simulink model "dual_arm_control"  (Simulink 7.8)
settings: Solver=ode1  StartTime=0.0  StopTime=inf  FixedStep=0.001  RelTol=1e-3
undefined symbols (not defined in the file): HIL
libraries: quarc_library x48, simulink x26, dspmtrx3 x5
(part 2 of 2)

== system dual_arm_control/Right Arm/contoller 22 ==
  qd : Inport
  q : Inport  Port=2
  en : Inport  Port=3
  Constant : Constant  Value=20
  Constant1 : Constant  Value=5e9
  Derivative3 : Derivative
  Derivative4 : Derivative
  Derivative5 : Derivative
  Memory3 : Memory  X0="[-0.0039    0.0394    0.0222   -0.2171]'"
  slotine's adaptive : MATLAB Function  TreatAsAtomicUnit=on
  tau : Outport
  ahat : Outport  Port=2
  wires:
  Derivative4/1 -> slotine's adaptive/6(qddotdot)
  Derivative5/1 -> slotine's adaptive/8(qdot)
  Derivative3/1 -> Derivative4/1, slotine's adaptive/5(qddot)
  slotine's adaptive/2(ahat) -> Memory3/1, ahat/1
  Memory3/1 -> slotine's adaptive/9(ahat_)
  Constant/1 -> slotine's adaptive/2(lambda)
  Constant1/1 -> slotine's adaptive/3(gamma)
  qd/1 -> slotine's adaptive/4(qd), Derivative3/1
  q/1 -> slotine's adaptive/7(q), Derivative5/1
  slotine's adaptive/1(tau) -> tau/1
  en/1 -> slotine's adaptive/1(en)

== system dual_arm_control/Right Arm/controller 21 ==
  qd : Inport
  q : Inport  Port=2
  en : Inport  Port=3
  Constant : Constant  Value=60
  Constant1 : Constant  Value=1e8
  Derivative3 : Derivative
  Derivative4 : Derivative
  Derivative5 : Derivative
  Memory3 : Memory  X0="[3.3914    0.1816    0.3172    0.1486   -5.6249]'"
  slotine's adaptive : MATLAB Function  TreatAsAtomicUnit=on
  tau : Outport
  ahat : Outport  Port=2
  wires:
  Derivative4/1 -> slotine's adaptive/6(qddotdot)
  Derivative5/1 -> slotine's adaptive/8(qdot)
  Derivative3/1 -> Derivative4/1, slotine's adaptive/5(qddot)
  slotine's adaptive/2(ahat) -> Memory3/1, ahat/1
  Memory3/1 -> slotine's adaptive/9(ahat_)
  Constant/1 -> slotine's adaptive/2(lambda)
  Constant1/1 -> slotine's adaptive/3(gamma)
  qd/1 -> slotine's adaptive/4(qd), Derivative3/1
  q/1 -> slotine's adaptive/7(q), Derivative5/1
  slotine's adaptive/1(tau) -> tau/1
  en/1 -> slotine's adaptive/1(en)

== system dual_arm_control/Right Arm/controller 23 ==
  qd : Inport
  q : Inport  Port=2
  en : Inport  Port=3
  Constant : Constant  Value=50
  Constant1 : Constant  Value=1e6
  Derivative3 : Derivative
  Derivative4 : Derivative
  Derivative5 : Derivative
  Memory3 : Memory  X0="[3.3916    0.1811    0.0907   -5.6122]'"
  slotine's adaptive : MATLAB Function  TreatAsAtomicUnit=on
  tau : Outport
  ahat : Outport  Port=2
  wires:
  Derivative4/1 -> slotine's adaptive/6(qddotdot)
  Derivative5/1 -> slotine's adaptive/8(qdot)
  Derivative3/1 -> Derivative4/1, slotine's adaptive/5(qddot)
  slotine's adaptive/2(ahat) -> Memory3/1, ahat/1
  Memory3/1 -> slotine's adaptive/9(ahat_)
  Constant/1 -> slotine's adaptive/2(lambda)
  Constant1/1 -> slotine's adaptive/3(gamma)
  qd/1 -> slotine's adaptive/4(qd), Derivative3/1
  q/1 -> slotine's adaptive/7(q), Derivative5/1
  slotine's adaptive/1(tau) -> tau/1
  en/1 -> slotine's adaptive/1(en)

== system dual_arm_control/Right Arm/controller 24 ==
  qd : Inport
  q : Inport  Port=2
  en : Inport  Port=3
  Constant : Constant  Value=50
  Constant1 : Constant  Value=1e6
  Derivative3 : Derivative
  Derivative4 : Derivative
  Derivative5 : Derivative
  Memory3 : Memory  X0="[0.0008    0.0273    0.0390   -0.0832]'"
  slotine's adaptive : MATLAB Function  TreatAsAtomicUnit=on
  tau : Outport
  ahat : Outport  Port=2
  wires:
  Derivative4/1 -> slotine's adaptive/6(qddotdot)
  Derivative5/1 -> slotine's adaptive/8(qdot)
  Derivative3/1 -> Derivative4/1, slotine's adaptive/5(qddot)
  slotine's adaptive/2(ahat) -> Memory3/1, ahat/1
  Memory3/1 -> slotine's adaptive/9(ahat_)
  Constant/1 -> slotine's adaptive/2(lambda)
  Constant1/1 -> slotine's adaptive/3(gamma)
  qd/1 -> slotine's adaptive/4(qd), Derivative3/1
  q/1 -> slotine's adaptive/7(q), Derivative5/1
  slotine's adaptive/1(tau) -> tau/1
  en/1 -> slotine's adaptive/1(en)

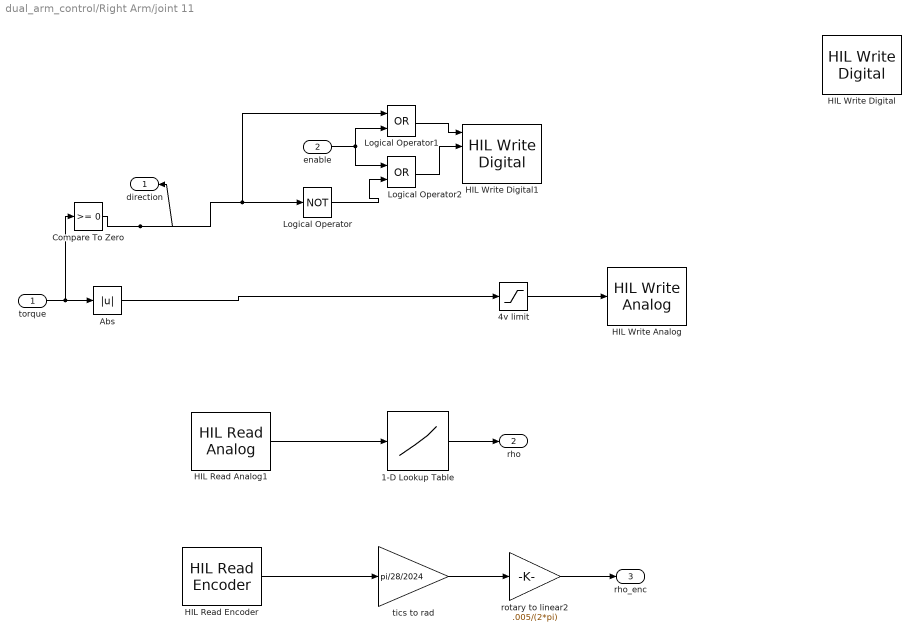
== system dual_arm_control/Right Arm/joint 11 ==
  torque : Inport
  enable : Inport  Port=2
  1-D Lookup Table : Lookup_n-D  NumberOfTableDimensions=1  BreakpointsForDimension1="[.147 .227 .277 .376 .459 .597  .742  .929  1.132  1.36 1.55   1.78  2.078 2.43 2.768  3.016   3.233  3.49  3.78  4.03 4.28]"  Table="[.04 .0375 .0357 .033 .031 .0286 .026  .022  .018  .015  .013  .01  .0088  .0077  .006   .005  .004  .003  .002  .001 0]"  RndMeth=Simplest  InputSameDT=on
  4v limit : Saturate  UpperLimit=4  LowerLimit=0
  Abs : Abs
  Compare To Zero : simulink/Logic and Bit Operations/Compare To Zero  relop=>=  OutDataTypeStr=boolean
  HIL Read Analog1 : quarc_library/Data Acquisition/Generic/Immediate I//O/HIL Read Analog  object_name=HIL-2  channels=[4]  sample_time=qc_get_step_size  active=on  vector_output=off
  HIL Read Encoder : quarc_library/Data Acquisition/Generic/Immediate I//O/HIL Read Encoder  object_name=HIL-2  channels=[0]  sample_time=qc_get_step_size  active=on  vector_output=off  data_type_mode=Inherit via back propagation  data_type=double
  HIL Write Analog : quarc_library/Data Acquisition/Generic/Immediate I//O/HIL Write Analog  object_name=HIL-1  channels=[0]  sample_time=-1  active=off  vector_input=off
  HIL Write Digital : quarc_library/Data Acquisition/Generic/Immediate I//O/HIL Write Digital  object_name=HIL-1  channels=[0:3]  sample_time=-1  active=off  vector_input=off
  HIL Write Digital1 : quarc_library/Data Acquisition/Generic/Immediate I//O/HIL Write Digital  object_name=HIL-1  channels=[40:43]  sample_time=-1  active=off  vector_input=off
  Logical Operator : Logic  Operator=NOT  AllPortsSameDT=off  OutDataTypeStr=boolean
  Logical Operator1 : Logic  Operator=OR  AllPortsSameDT=off  OutDataTypeStr=boolean
  Logical Operator2 : Logic  Operator=OR  AllPortsSameDT=off  OutDataTypeStr=boolean
  rotary to linear2 : Gain  Gain=.005/(2*pi)
  tics to rad : Gain  Gain=pi/28/2024
  direction : Outport
  rho : Outport  Port=2
  rho_enc : Outport  Port=3
  wires:
  4v limit/1 -> HIL Write Analog/1
  Compare To Zero/1 -> direction/1, Logical Operator/1, Logical Operator1/1
  Abs/1 -> 4v limit/1
  torque/1 -> Abs/1, Compare To Zero/1
  HIL Read Analog1/1 -> 1-D Lookup Table/1
  HIL Read Encoder/1 -> tics to rad/1
  Logical Operator/1 -> Logical Operator2/2
  enable/1 -> Logical Operator1/2, Logical Operator2/1
  Logical Operator1/1 -> HIL Write Digital1/1
  Logical Operator2/1 -> HIL Write Digital1/2
  1-D Lookup Table/1 -> rho/1
  tics to rad/1 -> rotary to linear2/1
  rotary to linear2/1 -> rho_enc/1

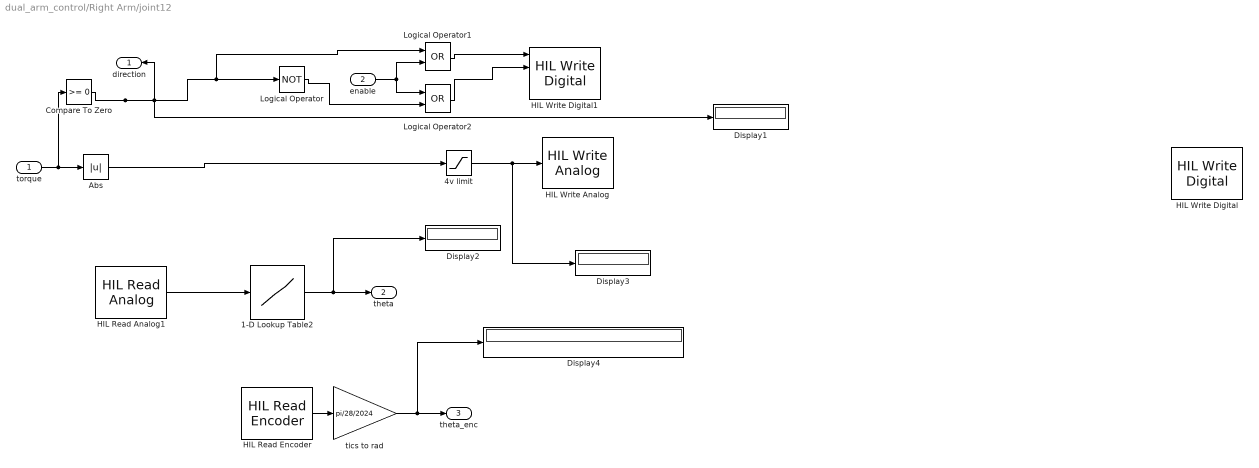
== system dual_arm_control/Right Arm/joint12 ==
  torque : Inport
  enable : Inport  Port=2
  1-D Lookup Table2 : Lookup_n-D  NumberOfTableDimensions=1  BreakpointsForDimension1=[.78 1.64 2.51 3.40 4.27]  Table=[2 1 0 -1 -2]  RndMeth=Simplest  InputSameDT=on
  4v limit : Saturate  UpperLimit=4  LowerLimit=0
  Abs : Abs
  Compare To Zero : simulink/Logic and Bit Operations/Compare To Zero  relop=>=  OutDataTypeStr=boolean
  Display{1..4} (4 alike) : Display
  HIL Read Analog1 : quarc_library/Data Acquisition/Generic/Immediate I//O/HIL Read Analog  object_name=HIL-1  channels=[3]  sample_time=qc_get_step_size  active=on  vector_output=off
  HIL Read Encoder : quarc_library/Data Acquisition/Generic/Immediate I//O/HIL Read Encoder  object_name=HIL-2  channels=[1]  sample_time=qc_get_step_size  active=on  vector_output=off  data_type_mode=Inherit via back propagation  data_type=double
  HIL Write Analog : quarc_library/Data Acquisition/Generic/Immediate I//O/HIL Write Analog  object_name=HIL-1  channels=[1]  sample_time=-1  active=off  vector_input=off
  HIL Write Digital : quarc_library/Data Acquisition/Generic/Immediate I//O/HIL Write Digital  object_name=HIL-1  channels=[4:7]  sample_time=-1  active=off  vector_input=off
  HIL Write Digital1 : quarc_library/Data Acquisition/Generic/Immediate I//O/HIL Write Digital  object_name=HIL-1  channels=[44:47]  sample_time=-1  active=off  vector_input=off
  Logical Operator : Logic  Operator=NOT  AllPortsSameDT=off  OutDataTypeStr=boolean
  Logical Operator1 : Logic  Operator=OR  AllPortsSameDT=off  OutDataTypeStr=boolean
  Logical Operator2 : Logic  Operator=OR  AllPortsSameDT=off  OutDataTypeStr=boolean
  tics to rad : Gain  Gain=pi/28/2024
  direction : Outport
  theta : Outport  Port=2
  theta_enc : Outport  Port=3
  wires:
  4v limit/1 -> HIL Write Analog/1, Display3/1
  Compare To Zero/1 -> Logical Operator/1, Logical Operator1/1, direction/1, Display1/1
  Abs/1 -> 4v limit/1
  torque/1 -> Abs/1, Compare To Zero/1
  HIL Read Analog1/1 -> 1-D Lookup Table2/1
  HIL Read Encoder/1 -> tics to rad/1
  Logical Operator1/1 -> HIL Write Digital1/1
  Logical Operator2/1 -> HIL Write Digital1/2
  Logical Operator/1 -> Logical Operator2/2
  enable/1 -> Logical Operator1/2, Logical Operator2/1
  tics to rad/1 -> theta_enc/1, Display4/1
  1-D Lookup Table2/1 -> Display2/1, theta/1

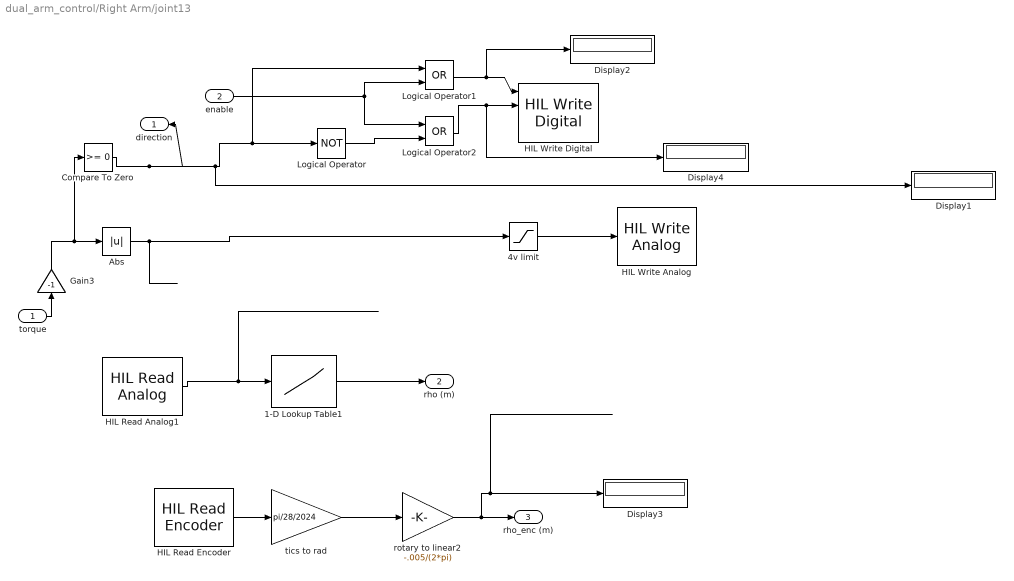
== system dual_arm_control/Right Arm/joint13 ==
  torque : Inport
  enable : Inport  Port=2
  1-D Lookup Table1 : Lookup_n-D  NumberOfTableDimensions=1  BreakpointsForDimension1="[.255 .369 .511 .661 .806 .966 1.075  1.274 1.456 1.643 1.858 2.075 2.328 2.50 2.753 3.011 3.23 3.39 4 4.191 4.384 4.628 4.84 4.963]"  Table=[0 .004 .0067 .0094 .012 .015 .017 .0199 .022 .0245 .0263 .0279 .0287 .0294 .030 .0315 .032 .034 .0357 .0365 .0373 .0385 .039 .04]+.001  RndMeth=Simplest  InputSameDT=on
  4v limit : Saturate  UpperLimit=4  LowerLimit=0
  Abs : Abs
  Compare To Zero : simulink/Logic and Bit Operations/Compare To Zero  relop=>=  OutDataTypeStr=boolean
  Display{1..4} (4 alike) : Display
  Gain3 : Gain  Gain=-1
  HIL Read Analog1 : quarc_library/Data Acquisition/Generic/Immediate I//O/HIL Read Analog  object_name=HIL-2  channels=[5]  sample_time=qc_get_step_size  active=on  vector_output=off
  HIL Read Encoder : quarc_library/Data Acquisition/Generic/Immediate I//O/HIL Read Encoder  object_name=HIL-2  channels=[2]  sample_time=qc_get_step_size  active=on  vector_output=off  data_type_mode=Inherit via back propagation  data_type=double
  HIL Write Analog : quarc_library/Data Acquisition/Generic/Immediate I//O/HIL Write Analog  object_name=HIL-1  channels=[2]  sample_time=-1  active=off  vector_input=off
  HIL Write Digital : quarc_library/Data Acquisition/Generic/Immediate I//O/HIL Write Digital  object_name=HIL-1  channels=[8:11]  sample_time=-1  active=off  vector_input=off
  Logical Operator : Logic  Operator=NOT  AllPortsSameDT=off  OutDataTypeStr=boolean
  Logical Operator1 : Logic  Operator=OR  AllPortsSameDT=off  OutDataTypeStr=boolean
  Logical Operator2 : Logic  Operator=OR  AllPortsSameDT=off  OutDataTypeStr=boolean
  rotary to linear2 : Gain  Gain=-.005/(2*pi)
  tics to rad : Gain  Gain=pi/28/2024
  direction : Outport
  rho (m) : Outport  Port=2
  rho_enc (m) : Outport  Port=3
  wires:
  4v limit/1 -> HIL Write Analog/1
  Compare To Zero/1 -> Logical Operator/1, Logical Operator1/1, Display1/1, direction/1
  Abs/1 -> 4v limit/1
  torque/1 -> Gain3/1
  HIL Read Analog1/1 -> 1-D Lookup Table1/1
  HIL Read Encoder/1 -> tics to rad/1
  Logical Operator/1 -> Logical Operator2/2
  Logical Operator2/1 -> HIL Write Digital/2, Display4/1
  Logical Operator1/1 -> HIL Write Digital/1, Display2/1
  enable/1 -> Logical Operator1/2, Logical Operator2/1
  1-D Lookup Table1/1 -> rho (m)/1
  tics to rad/1 -> rotary to linear2/1
  rotary to linear2/1 -> rho_enc (m)/1, Display3/1
  Gain3/1 -> Abs/1, Compare To Zero/1

== system dual_arm_control/Subsystem2/E1-1 ==
  Gain : Gain  Gain=pi
  HIL Read Analog : quarc_library/Data Acquisition/Generic/Immediate I//O/HIL Read Analog  object_name=HIL-2  channels=[0]  sample_time=qc_get_step_size  active=on  vector_output=off
  Out1 : Outport
  wires:
  HIL Read Analog/1 -> Gain/1
  Gain/1 -> Out1/1

== system dual_arm_control/Subsystem2/E1-2 ==
  Gain : Gain  Gain=pi
  HIL Read Analog : quarc_library/Data Acquisition/Generic/Immediate I//O/HIL Read Analog  object_name=HIL-2  channels=[1]  sample_time=qc_get_step_size  active=on  vector_output=off
  Out1 : Outport
  wires:
  HIL Read Analog/1 -> Gain/1
  Gain/1 -> Out1/1

== system dual_arm_control/Subsystem2/Subsystem ==
  DIR_1 : Inport
  EN_1 : Inport  Port=2
  PWM_1 : Inport  Port=3
  DIR_2 : Inport  Port=4
  EN_2 : Inport  Port=5
  PWM_2 : Inport  Port=6
  Constant3 : Constant
  Display : Display
  Display1 : Display
  E1-1 : Subsystem
  E1-2 : Subsystem
  E1-A : Subsystem
  Scope : Scope
  Scope1 : Scope
  wires:
  Constant3/1 -> E1-A/4(STBY)
  E1-1/1(IN1) -> E1-A/1(BIN1)
  E1-1/2(IN2) -> E1-A/2(BIN2)
  E1-1/3(PWM) -> E1-A/3(PWMB), Display/1, Scope/1
  E1-2/1(IN1) -> E1-A/5(AIN1)
  E1-2/2(IN2) -> E1-A/6(AIN2)
  E1-2/3(PWM) -> E1-A/7(PWMA), Display1/1, Scope1/1
  DIR_1/1 -> E1-1/1(DIR)
  EN_1/1 -> E1-1/2(EN)
  PWM_1/1 -> E1-1/3(DC)
  DIR_2/1 -> E1-2/1(DIR)
  EN_2/1 -> E1-2/2(EN)
  PWM_2/1 -> E1-2/3(DC)

== system dual_arm_control/IK_L/from omni/haptic gravity compensation ==
  position : Inport
  boundary force : Inport  Port=2
  status : Inport  Port=3
  Constant : Constant  Value=[0 0 .5]
  Derivative : Derivative
  Display1 : Display
  Display4 : Display
  Gain : Gain  Gain=-.030*diag([1 1 1])  Multiplication=Matrix(K*u)
  Gain1 : Gain  Gain=-.35*diag([1 1 1])  Multiplication=Matrix(K*u)
  Multiport Switch : MultiPortSwitch  Inputs=7  zeroidx=off
  Sum : Sum  Inputs=|+++++
  Sum1 : Sum  Inputs=|++
  force : Outport
  wires:
  Derivative/1 -> Gain/1
  Sum/1 -> force/1
  position/1 -> Derivative/1, Gain1/1
  Constant/1 -> Sum/4
  status/1 -> [status]
  Gain/1 -> Sum1/1
  Multiport Switch/1 -> Sum/1, Display4/1
  [status] -> Multiport Switch/1, Display1/1
  Sum1/1 -> Sum/5
  Gain1/1 -> Multiport Switch/7
  boundary force/1 -> Multiport Switch/8

== system dual_arm_control/IK_L/phantom/haptic gravity compensation ==
  position : Inport
  boundary force : Inport  Port=2
  status : Inport  Port=3
  Constant : Constant  Value=[0 0 .92]
  Derivative : Derivative
  Display1 : Display
  Display2 : Display
  Gain : Gain  Gain=-.1*diag([1 1 1])  Multiplication=Matrix(K*u)
  Gain1 : Gain  Gain=-.8*diag([1 1 1])  Multiplication=Matrix(K*u)
  Multiport Switch : MultiPortSwitch  Inputs=7  zeroidx=off
  Sum : Sum  Inputs=|+++++
  Sum1 : Sum  Inputs=|++
  force : Outport
  wires:
  Derivative/1 -> Gain/1
  Sum/1 -> force/1
  position/1 -> Derivative/1, Gain1/1
  Constant/1 -> Sum/4
  status/1 -> [status]
  Gain/1 -> Sum1/1
  Multiport Switch/1 -> Sum/1
  [status] -> Multiport Switch/1, Display1/1
  Sum1/1 -> Sum/5
  Gain1/1 -> Multiport Switch/7
  boundary force/1 -> Multiport Switch/8

== system dual_arm_control/Subsystem2/Subsystem/E1-1 ==
  DIR : Inport
  EN : Inport  Port=2
  DC : Inport  Port=3
  Logical Operator : Logic  AllPortsSameDT=off  OutDataTypeStr=boolean
  Logical Operator1 : Logic  AllPortsSameDT=off  OutDataTypeStr=boolean
  Logical Operator2 : Logic  Operator=NOT  AllPortsSameDT=off  OutDataTypeStr=boolean
  pwm generator : Subsystem
  IN1 : Outport
  IN2 : Outport  Port=2
  PWM : Outport  Port=3
  wires:
  Logical Operator2/1 -> Logical Operator/1
  DIR/1 -> Logical Operator2/1, Logical Operator1/1
  EN/1 -> Logical Operator/2, Logical Operator1/2
  Logical Operator/1 -> IN1/1
  Logical Operator1/1 -> IN2/1
  DC/1 -> pwm generator/1(In1)
  pwm generator/1(Out1) -> PWM/1

== system dual_arm_control/Subsystem2/Subsystem/E1-2 ==
  DIR : Inport
  EN : Inport  Port=2
  DC : Inport  Port=3
  Logical Operator : Logic  AllPortsSameDT=off  OutDataTypeStr=boolean
  Logical Operator1 : Logic  AllPortsSameDT=off  OutDataTypeStr=boolean
  Logical Operator2 : Logic  Operator=NOT  AllPortsSameDT=off  OutDataTypeStr=boolean
  pwm generator : Subsystem
  IN1 : Outport
  IN2 : Outport  Port=2
  PWM : Outport  Port=3
  wires:
  Logical Operator2/1 -> Logical Operator/1
  DIR/1 -> Logical Operator2/1, Logical Operator1/1
  EN/1 -> Logical Operator/2, Logical Operator1/2
  Logical Operator/1 -> IN1/1
  Logical Operator1/1 -> IN2/1
  DC/1 -> pwm generator/1(In1)
  pwm generator/1(Out1) -> PWM/1

== system dual_arm_control/Subsystem2/Subsystem/E1-A ==
  BIN1 : Inport
  BIN2 : Inport  Port=2
  PWMB : Inport  Port=3
  STBY : Inport  Port=4
  AIN1 : Inport  Port=5
  AIN2 : Inport  Port=6
  PWMA : Inport  Port=7
  HIL Write Digital : quarc_library/Data Acquisition/Generic/Immediate I//O/HIL Write Digital  object_name=HIL-2  channels=[44]  sample_time=-1  active=off  vector_input=off
  HIL Write Digital1 : quarc_library/Data Acquisition/Generic/Immediate I//O/HIL Write Digital  object_name=HIL-2  channels=[43]  sample_time=-1  active=off  vector_input=off
  HIL Write Digital2 : quarc_library/Data Acquisition/Generic/Immediate I//O/HIL Write Digital  object_name=HIL-2  channels=[42]  sample_time=-1  active=off  vector_input=off
  HIL Write Digital3 : quarc_library/Data Acquisition/Generic/Immediate I//O/HIL Write Digital  object_name=HIL-2  channels=[41]  sample_time=-1  active=off  vector_input=off
  HIL Write Digital4 : quarc_library/Data Acquisition/Generic/Immediate I//O/HIL Write Digital  object_name=HIL-2  channels=[45]  sample_time=-1  active=off  vector_input=off
  HIL Write Digital5 : quarc_library/Data Acquisition/Generic/Immediate I//O/HIL Write Digital  object_name=HIL-2  channels=[46]  sample_time=-1  active=off  vector_input=off
  HIL Write Digital6 : quarc_library/Data Acquisition/Generic/Immediate I//O/HIL Write Digital  object_name=HIL-2  channels=[47]  sample_time=-1  active=off  vector_input=off
  wires:
  BIN1/1 -> HIL Write Digital1/1
  BIN2/1 -> HIL Write Digital2/1
  PWMB/1 -> HIL Write Digital3/1
  STBY/1 -> HIL Write Digital/1
  AIN1/1 -> HIL Write Digital4/1
  AIN2/1 -> HIL Write Digital5/1
  PWMA/1 -> HIL Write Digital6/1

== system dual_arm_control/Subsystem2/Subsystem/E1-1/pwm generator ==
  In1 : Inport
  Counter Limited : simulink/Sources/Counter Limited  uplimit=10  tsamp=-1
  Gain : Gain  Gain=.1
  Relational Operator : RelationalOperator  Operator=<=  OutDataTypeStr=boolean
  Out1 : Outport
  wires:
  Counter Limited/1 -> Gain/1
  Gain/1 -> Relational Operator/1
  Relational Operator/1 -> Out1/1
  In1/1 -> Relational Operator/2

== system dual_arm_control/Subsystem2/Subsystem/E1-2/pwm generator ==
  In1 : Inport
  Counter Limited : simulink/Sources/Counter Limited  uplimit=10  tsamp=-1
  Gain : Gain  Gain=.1
  Relational Operator : RelationalOperator  Operator=<=  OutDataTypeStr=boolean
  Out1 : Outport
  wires:
  Counter Limited/1 -> Gain/1
  Gain/1 -> Relational Operator/1
  Relational Operator/1 -> Out1/1
  In1/1 -> Relational Operator/2

== matlab function Left Arm/controller 24/slotine's adaptive ==
  data: en input double; lambda input double; gamma input double; qd input double; qddot input double; qddotdot input double; q input double; tau output double; qdot input double; ahat output double; ahat_ input double
function [tau,ahat] = fcn(en,lambda,gamma,qd,qddot,qddotdot,q,qdot,ahat_)
%#codegen


qtilde=q-qd;
qtildedot=qdot-qddot;
s=qtildedot+lambda*qtilde;
Y=[qddotdot qddot sign(qdot) s ];
ahat=-.001*en/gamma*Y'*s+ahat_;
qr=qd-(ahat(end)+lambda)*qtilde;
qrdot=qddot-(ahat(end)+lambda)*qtilde;
qrdotdot=qddotdot-(ahat(end)+lambda)*qtildedot;

tau=[qrdotdot qrdot  sign(qdot) s ]*ahat;

== matlab function MATLAB Function ==
  data: ready_ input double; ready output double; status_ input double; delq_R_ input double; delq_L_ input double; status output double; delq_R output double; delq_L output double; dqin_L input double; dqin_R input double; time input double; dummy output double; qpot_R input double; qpot_L input double
function [ready,status,delq_R,delq_L,dummy] = fcn(ready_,status_,delq_R_,delq_L_,dqin_L,dqin_R,time,qpot_R,qpot_L)
%#codegen
dummy=0;
ready=ready_;
status=status_;
delq_R=delq_R_;
delq_L=delq_L_;
if time>2 && not(ready)
    
    switch status
        case 0
%             if time>2 && time<6
                if abs(qpot_L(2))<.1
                    status=1;
                end
                delq_L=[0 dqin_L(2) 0 0]';
                
%             end
        case 1
%             if time>6 && time<10
                
                if abs(qpot_L(1))<.001
                    status=2;
                end
                delq_L=[dqin_L(1) dqin_L(2) 0 0]';
                
%             end
        case 2
%             if time>10 && time<14
                
                if abs(qpot_L(3))<.001
                    status=3;
                end
                delq_L=[dqin_L(1) dqin_L(2) dqin_L(3) 0]';
                
%             end
        case 3
%             if time>14 && time<18
                if abs(qpot_R(2))<.1
                    status=4;
                end
                delq_R=[0 dqin_R(2) 0 0]';
                
%             end
        case 4
%             if time>18 && time<22
                
                if abs(qpot_R(1))<.001
                    status=5;
                end
                delq_R=[dqin_R(1) dqin_R(2) 0 0]';
                
%             end
        case 5
%             if time>22 && time<26
                
                if abs(qpot_R(3))<.001
                    status=6;

                end
                delq_R=[dqin_R(1) dqin_R(2) dqin_R(3) 0]';
                
%             end
        case 6 %match master and slave
            if time>20
                status=7;
                ready=1;
            end
    end
    
    
end

% if ready
%     delq_R=[dqin_R(1) 0 dqin_R(3) 0]';
%     delq_L=[dqin_L(1) 0 dqin_L(3) 0]';
% end

== matlab function filter/filter ==
  data: u input double; y output double; u_ input double
function y = fcn(u,u_)
%#codegen
if u>0
    a=2;
end
if abs(u-u_)<4*pi*.001
    y=u;
else
    y=u_+4*pi*.001*(u-u_)/abs(u-u_);

end

== matlab function Left Arm/controller 23/slotine's adaptive ==
  data: en input double; lambda input double; gamma input double; qd input double; qddot input double; qddotdot input double; q input double; tau output double; qdot input double; ahat output double; ahat_ input double
function [tau,ahat] = fcn(en,lambda,gamma,qd,qddot,qddotdot,q,qdot,ahat_)
%#codegen


qtilde=q-qd;
qtildedot=qdot-qddot;
s=qtildedot+lambda*qtilde;
Y=[qddotdot qddot sign(qdot) s ];
ahat=-.001*en/gamma*Y'*s+ahat_;
qr=qd-(ahat(end)+lambda)*qtilde;
qrdot=qddot-(ahat(end)+lambda)*qtilde;
qrdotdot=qddotdot-(ahat(end)+lambda)*qtildedot;

tau=[qrdotdot qrdot  sign(qdot) s ]*ahat;

== matlab function filter1/filter ==
  data: u input double; y output double; u_ input double
function y = fcn(u,u_)
%#codegen
if u>0
    a=2;
end
if abs(u-u_)<.02*.001
    y=u;
else
    y=u_+.02*.001*(u-u_)/abs(u-u_);

end

== matlab function Left Arm/contoller 22/slotine's adaptive ==
  data: en input double; lambda input double; gamma input double; qd input double; qddot input double; qddotdot input double; q input double; tau output double; qdot input double; ahat output double; ahat_ input double
function [tau,ahat] = fcn(en,lambda,gamma,qd,qddot,qddotdot,q,qdot,ahat_)
%#codegen


qtilde=q-qd;
qtildedot=qdot-qddot;
s=qtildedot+lambda*qtilde;
Y=[qddotdot qddot sign(qdot) s ];
ahat=-.001*en/gamma*Y'*s+ahat_;
qr=qd-(ahat(end)+lambda)*qtilde;
qrdot=qddot-(ahat(end)+lambda)*qtilde;
qrdotdot=qddotdot-(ahat(end)+lambda)*qtildedot;

tau=[qrdotdot qrdot  sign(qdot) s ]*ahat;

== matlab function filter2/filter ==
  data: u input double; y output double; u_ input double
function y = fcn(u,u_)
%#codegen
if u>0
    a=2;
end
if abs(u-u_)<4*pi*.001
    y=u;
else
    y=u_+4*pi*.001*(u-u_)/abs(u-u_);

end

== matlab function Left Arm/controller 21/slotine's adaptive ==
  data: en input double; lambda input double; gamma input double; qd input double; qddot input double; qddotdot input double; q input double; tau output double; qdot input double; ahat output double; ahat_ input double
function [tau,ahat] = fcn(en,lambda,gamma,qd,qddot,qddotdot,q,qdot,ahat_)
%#codegen


qtilde=q-qd;
qtildedot=qdot-qddot;
s=qtildedot+lambda*qtilde;
Y=[qddotdot qddot  sign(qdot)-1 sign(qdot)+1 s ];
ahat=-.001*en/gamma*Y'*s+ahat_;
qr=qd-(ahat(end)+lambda)*qtilde;
qrdot=qddot-(ahat(end)+lambda)*qtilde;
qrdotdot=qddotdot-(ahat(end)+lambda)*qtildedot;

tau=[qrdotdot qrdot sign(qdot)-1 sign(qdot)+1 s ]*ahat;

== matlab function filter3/filter ==
  data: u input double; y output double; u_ input double
function y = fcn(u,u_)
%#codegen
if u>0
    a=2;
end
if abs(u-u_)<.02*.001
    y=u;
else
    y=u_+.02*.001*(u-u_)/abs(u-u_);

end

== matlab function Right Arm/contoller 22/slotine's adaptive ==
  data: en input double; lambda input double; gamma input double; qd input double; qddot input double; qddotdot input double; q input double; tau output double; qdot input double; ahat output double; ahat_ input double
function [tau,ahat] = fcn(en,lambda,gamma,qd,qddot,qddotdot,q,qdot,ahat_)
%#codegen


qtilde=q-qd;
qtildedot=qdot-qddot;
s=qtildedot+lambda*qtilde;
Y=[qddotdot qddot sign(qdot) s ];
ahat=-.001*en/gamma*Y'*s+ahat_;
qr=qd-(ahat(end)+lambda)*qtilde;
qrdot=qddot-(ahat(end)+lambda)*qtilde;
qrdotdot=qddotdot-(ahat(end)+lambda)*qtildedot;

tau=[qrdotdot qrdot  sign(qdot) s ]*ahat;

== matlab function IK_L/IK_L/IK ==
  data: q_ input double; q output double; qm output double; qdot output double; p output double; pd input double; pd_d input double; F output double; k_ input double; k output double; r_ input double; r output double
function [q,qm,qdot,p,F,k,r] = fcn(q_,pd,pd_d,k_,r_)
%#codegen
kappa=1/8.5;
x=pd(1);
y=pd(2);
z=pd(3);
r=sqrt(x^2+y^2);

rho_1=q_(1);
theta_1=q_(2);
rho_2=q_(3);
%%%%%
J =...
    [ -kappa*cos(kappa*rho_1)*cos(theta_1)*(rho_1 - (rho_2+1)),   (sin(theta_1)*(cos(kappa*rho_1) - 1))/kappa + sin(kappa*rho_1)*sin(theta_1)*(rho_1 - (rho_2+1)), sin(kappa*rho_1)*cos(theta_1)
    -kappa*cos(kappa*rho_1)*sin(theta_1)*(rho_1 - (rho_2+1)), - (cos(theta_1)*(cos(kappa*rho_1) - 1))/kappa - sin(kappa*rho_1)*cos(theta_1)*(rho_1 - (rho_2+1)), sin(kappa*rho_1)*sin(theta_1)
    kappa*sin(kappa*rho_1)*(rho_1 - (rho_2+1)),                                                                                             0,              cos(kappa*rho_1)];


qdot=pinv(J)*pd_d;
p =...
    [ - (cos(theta_1)*(cos(kappa*rho_1) - 1))/kappa - sin(kappa*rho_1)*cos(theta_1)*(rho_1 - (rho_2+1))
    - (sin(theta_1)*(cos(kappa*rho_1) - 1))/kappa - sin(kappa*rho_1)*sin(theta_1)*(rho_1 - (rho_2+1))
    sin(kappa*rho_1)/kappa - cos(kappa*rho_1)*(rho_1 - (rho_2+1))];

%IK
theta_1_=theta_1;
theta_1=atan2(y,x);

if theta_1-theta_1_>3*pi/2
    k=k_-1;
elseif theta_1_-theta_1>3*pi/2
    k=k_+1;
else
    k=k_;
end
    
del=sqrt(abs(((1-kappa*sqrt(x^2+y^2))^2+kappa^2*z^2-1)/kappa^2));%del=rho_2-rho_1
rho_1=1/kappa*atan2(-(-kappa*z-(1-kappa*r)*kappa*-del),-kappa^2*z*-del+(1-kappa*r));
rho_2=rho_1+del-1;


if rho_2>=4
    rho_2=4;
elseif rho_2<=.1
    rho_2=.1;
end

if rho_2-rho_1<=0.1
    rho_1=rho_2-0.1;
end
if rho_1<=.1
    rho_1=.1;
end



q=[rho_1;theta_1;rho_2];
qm=[rho_1;theta_1+2*k*pi;rho_2];



% J_ =...
%     [ -kappa*cos(kappa*rho_1)*cos(theta_1)*(rho_1 - (rho_2+1)),   (sin(theta_1)*(cos(kappa*rho_1) - 1))/kappa + sin(kappa*rho_1)*sin(theta_1)*(rho_1 - (rho_2+1)), sin(kappa*rho_1)*cos(theta_1), 0
%     -kappa*cos(kappa*rho_1)*sin(theta_1)*(rho_1 - (rho_2+1)), - (cos(theta_1)*(cos(kappa*rho_1) - 1))/kappa - sin(kappa*rho_1)*cos(theta_1)*(rho_1 - (rho_2+1)), sin(kappa*rho_1)*sin(theta_1), 0
%     kappa*sin(kappa*rho_1)*(rho_1 - (rho_2+1)),                                                                                               0,              cos(kappa*rho_1), 0];




q=[rho_1;theta_1;rho_2];







%Force field barrier method
F=[0 0 0]';

if kappa*z<1
    s=asin(kappa*z)/kappa;
    if r>.95*(1-cos(kappa*s))/kappa
        F=(-.1-.1*abs(r-.95*(1-cos(kappa*s))/kappa))*[cos(theta_1)*cos(kappa*s);sin(theta_1)*cos(kappa*s);-sin(kappa*s)];
    end
end

== matlab function Right Arm/controller 21/slotine's adaptive ==
  data: en input double; lambda input double; gamma input double; qd input double; qddot input double; qddotdot input double; q input double; tau output double; qdot input double; ahat output double; ahat_ input double
function [tau,ahat] = fcn(en,lambda,gamma,qd,qddot,qddotdot,q,qdot,ahat_)
%#codegen


qtilde=q-qd;
qtildedot=qdot-qddot;
s=qtildedot+lambda*qtilde;
Y=[qddotdot qddot  sign(qdot)-1 sign(qdot)+1 s ];
ahat=-.001*en/gamma*Y'*s+ahat_;
qr=qd-(ahat(end)+lambda)*qtilde;
qrdot=qddot-(ahat(end)+lambda)*qtilde;
qrdotdot=qddotdot-(ahat(end)+lambda)*qtildedot;

tau=[qrdotdot qrdot sign(qdot)-1 sign(qdot)+1 s ]*ahat;

== matlab function Right Arm/controller 23/slotine's adaptive ==
  data: en input double; lambda input double; gamma input double; qd input double; qddot input double; qddotdot input double; q input double; tau output double; qdot input double; ahat output double; ahat_ input double
function [tau,ahat] = fcn(en,lambda,gamma,qd,qddot,qddotdot,q,qdot,ahat_)
%#codegen


qtilde=q-qd;
qtildedot=qdot-qddot;
s=qtildedot+lambda*qtilde;
Y=[qddotdot qddot sign(qdot) s ];
ahat=-.001*en/gamma*Y'*s+ahat_;
qr=qd-(ahat(end)+lambda)*qtilde;
qrdot=qddot-(ahat(end)+lambda)*qtilde;
qrdotdot=qddotdot-(ahat(end)+lambda)*qtildedot;

tau=[qrdotdot qrdot  sign(qdot) s ]*ahat;

== matlab function Right Arm/controller 24/slotine's adaptive ==
  data: en input double; lambda input double; gamma input double; qd input double; qddot input double; qddotdot input double; q input double; tau output double; qdot input double; ahat output double; ahat_ input double
function [tau,ahat] = fcn(en,lambda,gamma,qd,qddot,qddotdot,q,qdot,ahat_)
%#codegen


qtilde=q-qd;
qtildedot=qdot-qddot;
s=qtildedot+lambda*qtilde;
Y=[qddotdot qddot sign(qdot) s ];
ahat=-.001*en/gamma*Y'*s+ahat_;
qr=qd-(ahat(end)+lambda)*qtilde;
qrdot=qddot-(ahat(end)+lambda)*qtilde;
qrdotdot=qddotdot-(ahat(end)+lambda)*qtildedot;

tau=[qrdotdot qrdot  sign(qdot) s ]*ahat;

== matlab function filter4/filter ==
  data: u input double; y output double; u_ input double
function y = fcn(u,u_)
%#codegen
if u>0
    a=2;
end
if abs(u-u_)<4*pi*.001
    y=u;
else
    y=u_+4*pi*.001*(u-u_)/abs(u-u_);

end

== matlab function filter5/filter ==
  data: u input double; y output double; u_ input double
function y = fcn(u,u_)
%#codegen
if u>0
    a=2;
end
if abs(u-u_)<.02*.001
    y=u;
else
    y=u_+.02*.001*(u-u_)/abs(u-u_);

end

== matlab function filter6/filter ==
  data: u input double; y output double; u_ input double
function y = fcn(u,u_)
%#codegen
if u>0
    a=2;
end
if abs(u-u_)<4*pi*.001
    y=u;
else
    y=u_+4*pi*.001*(u-u_)/abs(u-u_);

end

== matlab function filter7/filter ==
  data: u input double; y output double; u_ input double
function y = fcn(u,u_)
%#codegen
if u>0
    a=2;
end
if abs(u-u_)<.02*.001
    y=u;
else
    y=u_+.02*.001*(u-u_)/abs(u-u_);

end

== matlab function IK_L/IK_R/IK ==
  data: q_ input double; q output double; qm output double; qdot output double; p output double; pd input double; pd_d input double; F output double; k_ input double; k output double; r_ input double; r output double
function [q,qm,qdot,p,F,k,r] = fcn(q_,pd,pd_d,k_,r_)
%#codegen
kappa=1/8.5;
x=pd(1);
y=pd(2);
z=pd(3);
r=sqrt(x^2+y^2);

rho_1=q_(1);
theta_1=q_(2);
rho_2=q_(3);
%%%%%
J =...
    [ -kappa*cos(kappa*rho_1)*cos(theta_1)*(rho_1 - (rho_2+1)),   (sin(theta_1)*(cos(kappa*rho_1) - 1))/kappa + sin(kappa*rho_1)*sin(theta_1)*(rho_1 - (rho_2+1)), sin(kappa*rho_1)*cos(theta_1)
    -kappa*cos(kappa*rho_1)*sin(theta_1)*(rho_1 - (rho_2+1)), - (cos(theta_1)*(cos(kappa*rho_1) - 1))/kappa - sin(kappa*rho_1)*cos(theta_1)*(rho_1 - (rho_2+1)), sin(kappa*rho_1)*sin(theta_1)
    kappa*sin(kappa*rho_1)*(rho_1 - (rho_2+1)),                                                                                             0,              cos(kappa*rho_1)];


qdot=pinv(J)*pd_d;
p =...
    [ - (cos(theta_1)*(cos(kappa*rho_1) - 1))/kappa - sin(kappa*rho_1)*cos(theta_1)*(rho_1 - (rho_2+1))
    - (sin(theta_1)*(cos(kappa*rho_1) - 1))/kappa - sin(kappa*rho_1)*sin(theta_1)*(rho_1 - (rho_2+1))
    sin(kappa*rho_1)/kappa - cos(kappa*rho_1)*(rho_1 - (rho_2+1))];

%IK
theta_1_=theta_1;
theta_1=atan2(y,x);

if theta_1-theta_1_>3*pi/2
    k=k_-1;
elseif theta_1_-theta_1>3*pi/2
    k=k_+1;
else
    k=k_;
end
    
del=sqrt(abs(((1-kappa*sqrt(x^2+y^2))^2+kappa^2*z^2-1)/kappa^2));%del=rho_2-rho_1
rho_1=1/kappa*atan2(-(-kappa*z-(1-kappa*r)*kappa*-del),-kappa^2*z*-del+(1-kappa*r));
rho_2=rho_1+del-1;


if rho_2>=4
    rho_2=4;
elseif rho_2<=.1
    rho_2=.1;
end

if rho_2-rho_1<=0.1
    rho_1=rho_2-0.1;
end
if rho_1<=.1
    rho_1=.1;
end



q=[rho_1;theta_1;rho_2];
qm=[rho_1;theta_1+2*k*pi;rho_2];



% J_ =...
%     [ -kappa*cos(kappa*rho_1)*cos(theta_1)*(rho_1 - (rho_2+1)),   (sin(theta_1)*(cos(kappa*rho_1) - 1))/kappa + sin(kappa*rho_1)*sin(theta_1)*(rho_1 - (rho_2+1)), sin(kappa*rho_1)*cos(theta_1), 0
%     -kappa*cos(kappa*rho_1)*sin(theta_1)*(rho_1 - (rho_2+1)), - (cos(theta_1)*(cos(kappa*rho_1) - 1))/kappa - sin(kappa*rho_1)*cos(theta_1)*(rho_1 - (rho_2+1)), sin(kappa*rho_1)*sin(theta_1), 0
%     kappa*sin(kappa*rho_1)*(rho_1 - (rho_2+1)),                                                                                               0,              cos(kappa*rho_1), 0];




q=[rho_1;theta_1;rho_2];







%Force field barrier method
F=[0 0 0]';

if kappa*z<1
    s=asin(kappa*z)/kappa;
    if r>.97*(1-cos(kappa*s))/kappa
        F=(-.1-.1*abs(r-.97*(1-cos(kappa*s))/kappa))*[cos(theta_1)*cos(kappa*s);sin(theta_1)*cos(kappa*s);-sin(kappa*s)];
    end
end

== matlab function Left Arm/MATLAB Function ==
  data: theta_pot input double; theta_enc input double; theta_ input double; theta output double; error_ input double; error output double
function [theta,error] = fcn(theta_pot,theta_enc,theta_,error_)
%#codegen



if -1.3<atan2(sin(theta_),cos(theta_)) && atan2(sin(theta_),cos(theta_))<1.3
    
    error=theta_pot-atan2(sin(theta_enc),cos(theta_enc));
    
else
    error=error_;
end

theta=theta_enc+error;

== matlab function Subsystem2/MATLAB Function ==
  data: u input double; dir output double; en output double; pos input double; pwm output double; pmax input double; pmin input double
function [dir,en,pwm] = fcn(u,pos,pmax,pmin)
%#codegen

% en=1;
% dir=1;
% pwm=.5;
% switch u
%     case 0
%         en=0;
%         dir=1;
%     case 1%open
%         en=1;
%         dir=1;
%     case 2%close
%         en=1;
%         dir=0;
% 
% end
% 
% 
en=1;
dir=1;
pwm=.7;

if u>0 
    dir=0;%close
else
    dir=1;
end
if pos>pmax && dir==1
    en=0;
end
if pos<pmin && dir==0
    en=0;
end

== matlab function Subsystem2/MATLAB Function1 ==
  data: u input double; dir output double; en output double; pos input double; pwm output double; pmax input double; pmin input double
function [dir,en,pwm] = fcn(u,pos,pmax,pmin)
%#codegen

% en=1;
% dir=1;
% pwm=.6;
% switch u
%     case 0
%         en=0;
%         dir=1;
%     case 1%open
%         en=1;
%         dir=1;
%     case 2%close
%         en=1;
%         dir=0;
% 
% end


en=1;
dir=1;
pwm=.9;

if u>0 
    dir=1;%close
else
    dir=0;
end



if pos<pmin && dir==1
    en=0;
end
if pos>pmax && dir==0
    en=0;
end
